simulink model "task"  (Simulink 3.00)
libraries: mathlib x8, logiclib x1, execlib x1, reglib x1, analoglib x1

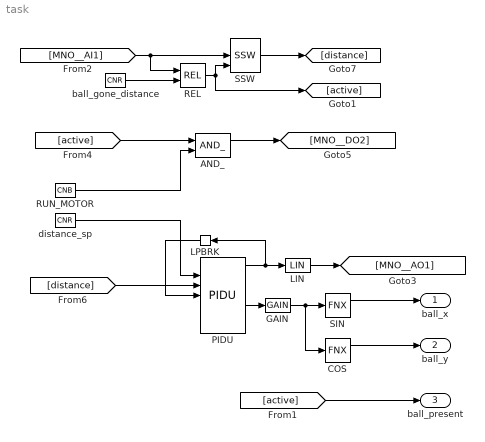
== system task ==
  AND_ : logiclib/AND_
  COS : mathlib/FNX  ifn=5: cos  yerr=0
  GAIN : mathlib/GAIN  k=0.12036
  LIN : mathlib/LIN  u1=-1  y1=0  u2=1  y2=5
  LPBRK : execlib/LPBRK  Orientation=left
  PIDU : reglib/PIDU  irtype=5: PD  RACT=on  k=0.15  ti=4  td=0.001  nd=2  b=1  c=0  tt=1  hilim=0.08  lolim=-0.08  dz=0  icotype=1: Analog
  REL : mathlib/REL  irel=4: greater than (>)
  RUN_MOTOR : mathlib/CNB  YCN=on
  SIN : mathlib/FNX  ifn=14: sin  yerr=0
  SSW : analoglib/SSW
  ball_gone_distance : mathlib/CNR  ycn=0.5
  distance_sp : mathlib/CNR  ycn=3.16
  ball_x : Outport  Port=1
  ball_y : Outport  Port=2
  ball_present : Outport  Port=3
  wires:
  AND_/1 -> [MNO__DO2]
  COS/1 -> ball_y/1
  [active] -> ball_present/1
  [MNO__AI1] -> REL/1, SSW/2
  [active] -> AND_/1
  [distance] -> PIDU/3
  GAIN/1 -> COS/1, SIN/1
  LIN/1 -> [MNO__AO1]
  LPBRK/1 -> PIDU/4
  PIDU/1 -> LIN/1, LPBRK/1
  PIDU/3 -> GAIN/1
  REL/1 -> [active], SSW/3
  RUN_MOTOR/1 -> AND_/2
  SIN/1 -> ball_x/1
  SSW/1 -> [distance]
  ball_gone_distance/1 -> REL/2
  distance_sp/1 -> PIDU/2
